simulink model "lechape_ex1_simu2016"  (Simulink 8.7)
settings: Solver=VariableStepAuto  SolverMode=SingleTasking  StartTime=0.0  StopTime=Tsim  RelTol=1e-3
values from neighbouring files (symbols this model uses):
  A = [0 1; -9 3]    [lechape_ex1_code.m]    (also in lechape_ex2_code.m)
  B = [0 1]'    [lechape_ex1_code.m]    (also in lechape_ex2_code.m)
  h = 0.5    [lechape_ex1_code.m]    (also in lechape_ex2_code.m)
  kd = 18    [lechape_ex1_code.m]
  ki = 60    [lechape_ex1_code.m]
  kp = 45    [lechape_ex1_code.m]
  N = 500    [lechape_ex1_code.m]    (also in lechape_ex2_code.m)
  x0_artstein = [1.5 -23]'    [lechape_ex1_code.m]
  x0_lechappe = [1.5 -23]'    [lechape_ex1_code.m]
undefined symbols (not defined in the file or in its folder): Ad, Bd, Cd, Dd, KSoma, Q, tal
settings Model: Creator=Vasco  LastModifiedBy=Vasco
settings DataIOCC: LimitDataPoints=off  SaveFormat=Dataset
settings DebuggingCC: UnderspecifiedInitializationDetection=Simplified  MergeDetectMultiDrivingBlocksExec=error  UnconnectedInputMsg=none  UnconnectedOutputMsg=none  UnconnectedLineMsg=none  SFUnexpectedBacktrackingDiag=error  SFNoUnconditionalDefaultTransitionDiag=error
settings HardwareCC: ProdBitPerPointer=64  ProdLargestAtomicFloat=Float  ProdIntDivRoundTo=Zero  ProdEndianess=LittleEndian  ProdWordSize=64  ProdHWDeviceType=Intel->x86-64 (Windows64)
settings ModelReferenceCC: EnableRefExpFcnMdlSchedulingChecks=off  PropagateSignalLabelsOutOfModel=on
settings SFSimCC: SimUseLocalCustomCode=on
settings RTWCC: RTWUseLocalCustomCode=on
settings GRTTargetCC: TargetLangStandard=C99 (ISO)
settings ConfigComp: CovMetricSettings=dwe  CovSaveCumulativeToWorkspaceVar=off  CovSaveSingleToWorkspaceVar=off  CovModelRefEnable=off  CovExternalEMLEnable=on

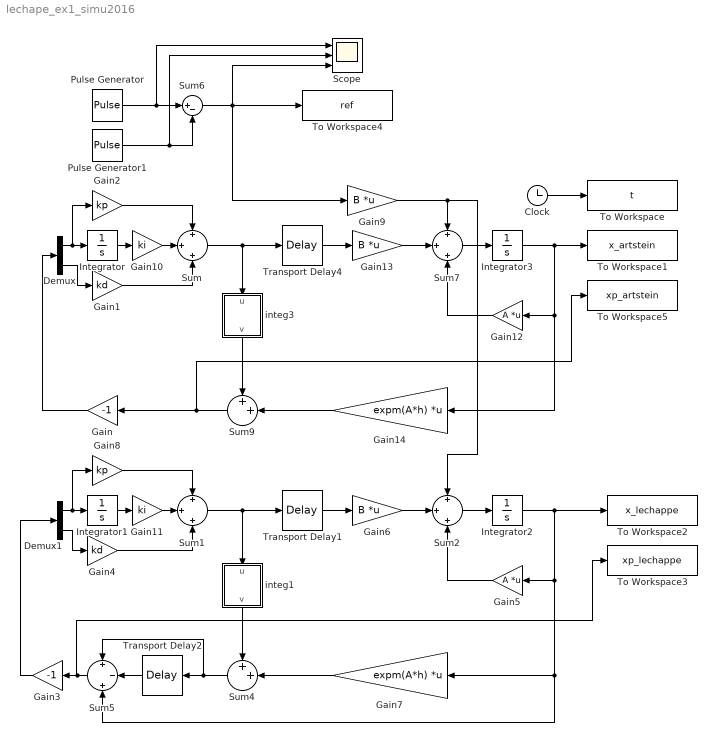
== system lechape_ex1_simu2016 ==
  Clock : Clock
  Demux : Demux  Outputs=2
  Demux1 : Demux  Outputs=2
  Gain : Gain  Gain=-1
  Gain1 : Gain  Gain=kd
  Gain10 : Gain  Gain=ki
  Gain11 : Gain  Gain=ki
  Gain12 : Gain  Gain=A  Multiplication=Matrix(K*u)
  Gain13 : Gain  Gain=B  Multiplication=Matrix(K*u)
  Gain14 : Gain  Gain=expm(A*h)  Multiplication=Matrix(K*u)
  Gain2 : Gain  Gain=kp
  Gain3 : Gain  Gain=-1
  Gain4 : Gain  Gain=kd
  Gain5 : Gain  Gain=A  Multiplication=Matrix(K*u)
  Gain6 : Gain  Gain=B  Multiplication=Matrix(K*u)
  Gain7 : Gain  Gain=expm(A*h)  Multiplication=Matrix(K*u)
  Gain8 : Gain  Gain=kp
  Gain9 : Gain  Gain=B  Multiplication=Matrix(K*u)
  Integrator : Integrator
  Integrator1 : Integrator
  Integrator2 : Integrator  InitialCondition=x0_lechappe
  Integrator3 : Integrator  InitialCondition=x0_artstein
  Pulse Generator : DiscretePulseGenerator  PulseType=Time based  Amplitude=4.5  Period=20  PulseWidth=25  PhaseDelay=5.5
  Pulse Generator1 : DiscretePulseGenerator  PulseType=Time based  Amplitude=4.5  Period=20  PulseWidth=25  PhaseDelay=15.5
  Scope : Scope  NumInputPorts=3
  Sum{,1..2,7} (4 alike) : Sum  Inputs=+|+|+
  Sum4 : Sum  Inputs=++|
  Sum5 : Sum  Inputs=+|-|+
  Sum6 : Sum  Inputs=|+-
  Sum9 : Sum  Inputs=++|
  To Workspace : ToWorkspace  VariableName=t  SampleTime=-1
  To Workspace1 : ToWorkspace  VariableName=x_artstein  SampleTime=-1
  To Workspace2 : ToWorkspace  VariableName=x_lechappe  SampleTime=-1
  To Workspace3 : ToWorkspace  VariableName=xp_lechappe  SampleTime=-1
  To Workspace4 : ToWorkspace  VariableName=ref  SampleTime=-1
  To Workspace5 : ToWorkspace  VariableName=xp_artstein  SampleTime=-1
  Transport Delay1 : TransportDelay  DelayTime=h
  Transport Delay2 : TransportDelay  DelayTime=h
  Transport Delay4 : TransportDelay  DelayTime=h
  integ1 : Subsystem
  integ3 : Subsystem
  wires:
  Clock/1 -> To Workspace/1
  integ3/1(v) -> Sum9/1
  Gain13/1 -> Sum7/2
  Gain12/1 -> Sum7/3
  Sum7/1 -> Integrator3/1
  Transport Delay4/1 -> Gain13/1
  Sum9/1 -> To Workspace5/1, Gain/1
  Gain14/1 -> Sum9/2
  Sum/1 -> Transport Delay4/1, integ3/1(u)
  Gain/1 -> Demux/1
  Integrator3/1 -> Gain14/1, Gain12/1, To Workspace1/1
  Demux/2 -> Gain1/1
  Integrator/1 -> Gain10/1
  Gain1/1 -> Sum/3
  Demux/1 -> Gain2/1, Integrator/1
  Gain2/1 -> Sum/1
  Gain4/1 -> Sum1/3
  Gain8/1 -> Sum1/1
  Demux1/1 -> Gain8/1, Integrator1/1
  Gain3/1 -> Demux1/1
  Demux1/2 -> Gain4/1
  Gain5/1 -> Sum2/3
  integ1/1(v) -> Sum4/1
  Sum1/1 -> Transport Delay1/1, integ1/1(u)
  Sum2/1 -> Integrator2/1
  Gain7/1 -> Sum4/2
  Gain6/1 -> Sum2/2
  Integrator2/1 -> Sum5/3, Gain7/1, Gain5/1, To Workspace2/1
  Integrator1/1 -> Gain11/1
  Transport Delay1/1 -> Gain6/1
  Sum5/1 -> Gain3/1, To Workspace3/1
  Sum4/1 -> Transport Delay2/1, Sum5/1
  Transport Delay2/1 -> Sum5/2
  Pulse Generator/1 -> Scope/1, Sum6/1
  Pulse Generator1/1 -> Scope/2, Sum6/2
  Gain9/1 -> Sum2/1, Sum7/1
  Gain10/1 -> Sum/2
  Gain11/1 -> Sum1/2
  Sum6/1 -> Scope/3, Gain9/1, To Workspace4/1

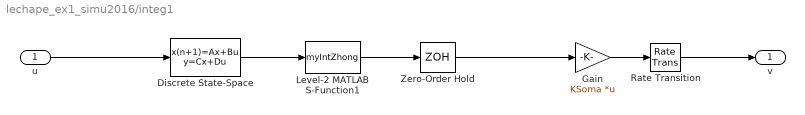
== system lechape_ex1_simu2016/integ1 ==
  u : Inport
  Discrete State-Space : DiscreteStateSpace  A=Ad  B=Bd  C=Cd  D=Dd  SampleTime=tal
  Gain : Gain  Gain=KSoma  Multiplication=Matrix(K*u)
  Level-2 MATLAB S-Function1 : M-S-Function  FunctionName=myIntZhong  Parameters=tal,A,B,Q,N
  Rate Transition : RateTransition
  Zero-Order Hold : ZeroOrderHold  SampleTime=tal
  v : Outport
  wires:
  Rate Transition/1 -> v/1
  u/1 -> Discrete State-Space/1
  Gain/1 -> Rate Transition/1
  Zero-Order Hold/1 -> Gain/1
  Discrete State-Space/1 -> Level-2 MATLAB S-Function1/1
  Level-2 MATLAB S-Function1/1 -> Zero-Order Hold/1

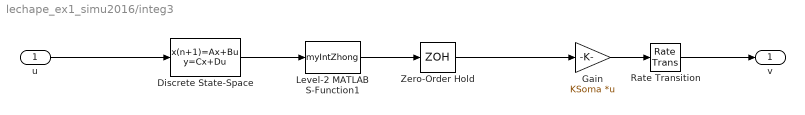
== system lechape_ex1_simu2016/integ3 ==
  u : Inport
  Discrete State-Space : DiscreteStateSpace  A=Ad  B=Bd  C=Cd  D=Dd  SampleTime=tal
  Gain : Gain  Gain=KSoma  Multiplication=Matrix(K*u)
  Level-2 MATLAB S-Function1 : M-S-Function  FunctionName=myIntZhong  Parameters=tal,A,B,Q,N
  Rate Transition : RateTransition
  Zero-Order Hold : ZeroOrderHold  SampleTime=tal
  v : Outport
  wires:
  Rate Transition/1 -> v/1
  u/1 -> Discrete State-Space/1
  Gain/1 -> Rate Transition/1
  Zero-Order Hold/1 -> Gain/1
  Discrete State-Space/1 -> Level-2 MATLAB S-Function1/1
  Level-2 MATLAB S-Function1/1 -> Zero-Order Hold/1
